simulink model "RCCircuit"  (R2013b)
settings: Solver=ode45  StartTime=0.0  StopTime=10  RelTol=1e-3
undefined symbols (not defined in the file or in its folder): C, R
settings Model: Creator=gyurse  LastModifiedBy=gyurse
settings ConfigurationSet: Description=SimMechanics 2G

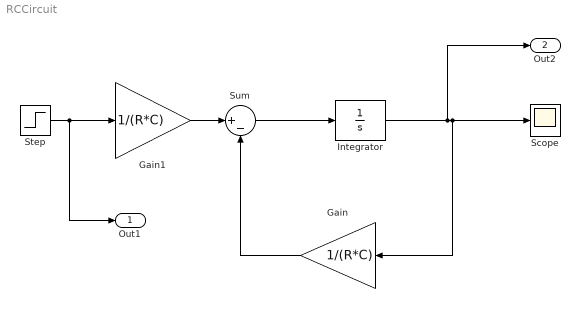
== system RCCircuit ==
  Gain : Gain  Gain=1/(R*C)
  Gain1 : Gain  Gain=1/(R*C)
  Integrator : Integrator
  Scope : Scope
  Step : Step  Time=0  SampleTime=0
  Sum : Sum  Inputs=|+-
  Out1 : Outport
  Out2 : Outport  Port=2
  wires:
  Sum/1 -> Integrator/1
  Integrator/1 -> Out2/1, Gain/1, Scope/1
  Gain/1 -> Sum/2
  Gain1/1 -> Sum/1
  Step/1 -> Out1/1, Gain1/1
